simulink model "uplink_4c1r"  (Simulink 8.7)
settings: Solver=VariableStepDiscrete  StartTime=0.0  StopTime=DDC_Lineup_param.endTime  RelTol=1e-3
PreLoadFcn:
  | % Run the setup script when the model is opened
  | setup_uplink_4c1r;
InitFcn:
  | % Run the setup script again just before the
  | % model is run, so that any updates made
  | % after opening are applied.
  | setup_uplink_4c1r;
  | %% DSPBuilder Start
  | alt_dspbuilder_update_model(bdroot)
  | %% DSPBuilder End
undefined symbols (not defined in the file or in its folder): AdvDSPBChannelOutDisplay, carrier_separation, DDC_Lineup_param, dpoly, dspba_ChannelInVis, dspba_ChannelOutVis, dspba_internal_get_channel_ports, dspba_internal_get_demux_ports, evalAionMaskParam, latency, Power_Meter, primtype, Subsystem, uplink_4c1r_carrier_seperation_4c, uplink_4c1r_pd_accu_reg_block, uplink_4c1r_power_meter_1carrier, value
undefined symbols (not defined in the file): power_meter_param
libraries: DSPBAPrim x119, DSPBABase x26, uplink_4c1r_pipereg_lib x22, DSPBAModelBus x9, DSPBAFilters x5, uplink_4c1r_register x5, uplink_4c1r_accumulator x5, uplink_4c1r_peak_detector x5, uplink_4c1r_iq_square x4, DSPBAControl x2, DSPBAWaveformSynth x2, DSPBAUtilities x1
(part 1 of 3)
Description:
  | DSP Builder Advanced Template for Template Design implementing ModelIP designs
settings Model: Creator=mjervis  LastModifiedBy=5g
settings DataIOCC: SignalLoggingSaveFormat=ModelDataLogs
settings OptimizationCC: ExpressionDepthLimit=2147483647
settings DebuggingCC: SolverPrmCheckMsg=warning  InheritedTsInSrcMsg=none  IntegerOverflowMsg=none  FcnCallInpInsideContextMsg=UseLocalSettings  StateNameClashWarn=warning  IntegerSaturationMsg=none
settings GRTTargetCC: CombineOutputUpdateFcns=off  GRTInterface=on

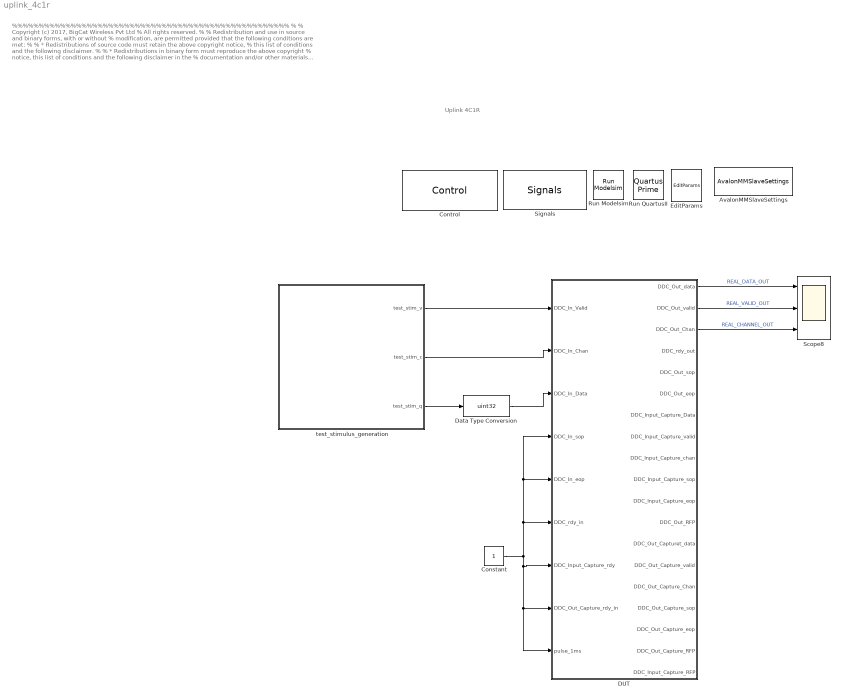
== system uplink_4c1r ==
  note: %%%%%%%%%%%%%%%%%%%%%%%%%%%%%%%%%%%%%%%%%%%%%%%%%%%%
      |  %
      |  % Copyright (c) 2017, BigCat Wireless Pvt Ltd
      |  % All rights reserved.
      |  %
      |  % Redistribution and use in source and binary forms, with or without
      |  % modification, are permitted provided that the following conditions are met:
      |  %
      |  %     * Redistributions of source code must retain the above copyright notice,
      |  %       this list of conditions and the following disclaimer.
      |  %
      |  %     * Redistributions in binary form must reproduce the above copyright
      |  %       notice, this list of conditions and the following disclaimer in the
      |  %       documentation and/or other materials provided with the distribution.
      |  %
      |  %     * Neither the name of the copyright holder nor the names of its contributors
      |  %       may be used to endorse or promote products derived from this software
      |  %       without specific prior written permission.
      |  %
      |  %
      |  %
      |  % THIS SOFTWARE IS PROVIDED BY THE COPYRIGHT HOLDERS AND CONTRIBUTORS "AS IS"
      |  % AND ANY EXPRESS OR IMPLIED WARRANTIES, INCLUDING, BUT NOT LIMITED TO, THE
      |  % IMPLIED WARRANTIES OF MERCHANTABILITY AND FITNESS FOR A PARTICULAR PURPOSE ARE
      |  % DISCLAIMED. IN NO EVENT SHALL THE COPYRIGHT HOLDER OR CONTRIBUTORS BE LIABLE
      |  % FOR ANY DIRECT, INDIRECT, INCIDENTAL, SPECIAL, EXEMPLARY, OR CONSEQUENTIAL
      |  % DAMAGES (INCLUDING, BUT NOT LIMITED TO, PROCUREMENT OF SUBSTITUTE GOODS OR
      |  % SERVICES; LOSS OF USE, DATA, OR PROFITS; OR BUSINESS INTERRUPTION) HOWEVER
      |  % CAUSED AND ON ANY THEORY OF LIABILITY, WHETHER IN CONTRACT, STRICT LIABILITY,
      |  % OR TORT (INCLUDING NEGLIGENCE OR OTHERWISE) ARISING IN ANY WAY OUT OF THE USE
      |  % OF THIS SOFTWARE, EVEN IF ADVISED OF THE POSSIBILITY OF SUCH DAMAGE.
      |  %
      |   %%%%%%%%%%%%%%%%%%%%%%%%%%%%%%%%%%%%%%%%%%%%%%%%%%%%%
  note: Uplink 4C1R
  AvalonMMSlaveSettings : DSPBABase/AvalonMMSlaveSettings
  Constant : Constant  OutDataTypeStr=boolean
  Control : DSPBABase/Control  generate=on  language=VHDL  destination=./rtl  destination_gui=./rtl  make_full_path=off  path_is_relative=on  autotestbench=off  signaldepth=2  coveragetestbench=on  logs=off  spacewidth=2  spacenum=1  addrwidth=10  datawidth=32  dataendian=Big Endian  hierarchicalnames=off  ramThresholdBits=-1  distRamThresholdBits=-1  mlabThresholdBits=-1  hardMultiplierThresholdLuts=-1  version=20090407  errorOnChanMismatch=1  errorOnGPIOMismatch=0  importModelsimResults=0  cycleAccurate=off  reinterpretCastMult=off  paramFile=uplink_4c1r_params.xml
  DUT : Subsystem
  Data Type Conversion : DataTypeConversion  OutDataTypeStr=uint32
  EditParams : DSPBABase/EditParams  version=20090407
  Run Modelsim : DSPBABase/Run Modelsim  version=20090407
  "Run QuartusII " : DSPBABase/Quartus Prime  version=20090407
  Scope8 : Scope  NumInputPorts=3
  Signals : DSPBABase/Signals  clk=clk  freq=DDC_Lineup_param.ClockRate  margin=DDC_Lineup_param.ClockMargin  rst=areset  rstactive=High  bus=bus  enbusclock=on  busfreq=DDC_Lineup_param.ClockRate/10  bussync=on  version=20090407
  test_stimulus_generation : Subsystem
  wires:
  test_stimulus_generation/3(test_stim_q) -> Data Type Conversion/1
  DUT/1(DDC_Out_data) -> Scope8/1  "REAL_DATA_OUT"
  Constant/1 -> DUT/7(DDC_Input_Capture_rdy), DUT/8(DDC_Out_Capture_rdy_in), DUT/9(pulse_1ms), DUT/5(DDC_In_eop), DUT/4(DDC_In_sop), DUT/6(DDC_rdy_in)
  Data Type Conversion/1 -> DUT/3(DDC_In_Data)
  test_stimulus_generation/2(test_stim_c) -> DUT/2(DDC_In_Chan)
  test_stimulus_generation/1(test_stim_v) -> DUT/1(DDC_In_Valid)
  DUT/2(DDC_Out_valid) -> Scope8/2  "REAL_VALID_OUT"
  DUT/3(DDC_Out_Chan) -> Scope8/3  "REAL_CHANNEL_OUT"

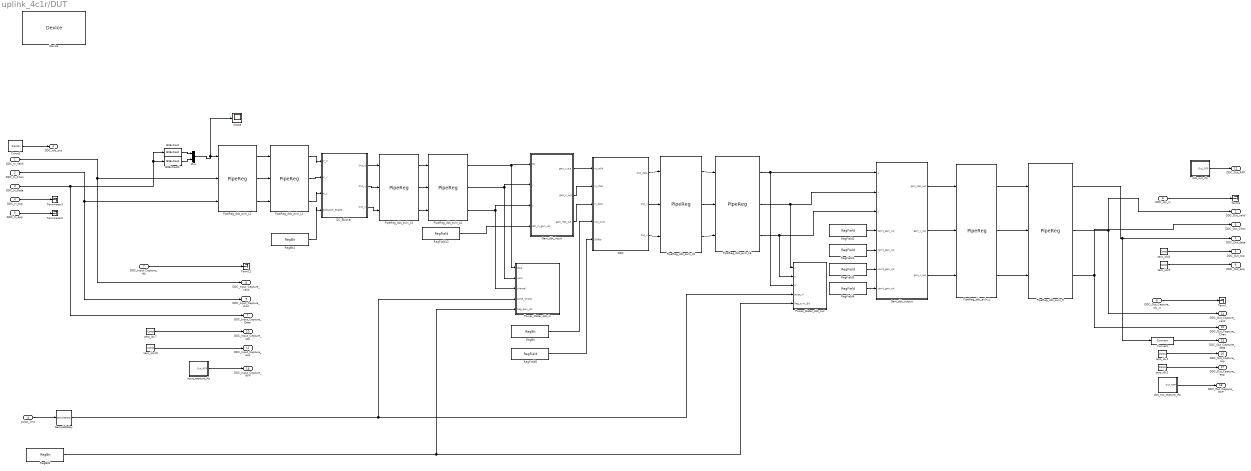
== system uplink_4c1r/DUT ==
  DDC_In_Valid : Inport
  DDC_In_Chan : Inport  Port=2
  DDC_In_Data : Inport  Port=3
  DDC_In_sop : Inport  Port=4  OutDataTypeStr=boolean
  DDC_In_eop : Inport  Port=5  OutDataTypeStr=boolean
  DDC_rdy_in : Inport  Port=6  OutDataTypeStr=boolean
  DDC_Input_Capture_rdy : Inport  Port=7  OutDataTypeStr=boolean
  DDC_Out_Capture_rdy_in : Inport  Port=8  OutDataTypeStr=boolean
  pulse_1ms : Inport  Port=9
  BitExtract : DSPBAPrim/BitExtract  primtype=bitextract  nInputs=1  nOutputs=1  omode=Specify via dialog  otype=sfix(16)  scale=2^-15  rndmethod=Unbiased  factor=1  satmethod=Symmetric  shift_vec=[0 1 2 -1]  value=0  inPortNames=[' '; ' ';]  outPortNames=[' ']  dspbaimage=dspba_prim.jpg  text=fprintf('..%d', value);  style=Optimised  visibilities=8+1024  version=20090407
  BitExtract1 : DSPBAPrim/BitExtract  primtype=bitextract  nInputs=1  nOutputs=1  omode=Specify via dialog  otype=sfix(16)  scale=2^-15  rndmethod=Unbiased  factor=1  satmethod=Symmetric  shift_vec=[0 1 2 -1]  value=16  inPortNames=[' '; ' ';]  outPortNames=[' ']  dspbaimage=dspba_prim.jpg  text=fprintf('..%d', value);  style=Optimised  visibilities=8+1024  version=20090407
  Const2 : DSPBAPrim/Const  primtype=const  nInputs=0  nOutputs=1  omode=boolean  otype=sfix(16)  scale=2^-15  rndmethod=Unbiased  factor=1  satmethod=Symmetric  shift_vec=[0 1 2 -1]  value=1  inPortNames=['+'; '+';]  outPortNames=[' ']  dspbaimage=dspba_prim.jpg  text=fprintf('%s', num2str(value));  style=Optimised  visibilities=8 + 1024  floatPrecision=float32_m23  version=20120820
  Convert : DSPBAPrim/Convert  primtype=convert  nInputs=1  nOutputs=1  omode=Specify via dialog  otype=sfix(32)  scale=2^-31  rndmethod=Unbiased  factor=1  satmethod=None  shift_vec=[0 1 2 -1]  value=round([0:255]/17)  inPortNames=[' '; ' ';]  outPortNames=[' '; 'c']  dspbaimage=dspba_prim.jpg  text=fprintf('convert');  style=Optimised  visibilities=8+64+256+2^17  clipdetect=off  floatPrecision=float32_m23  advOptions=[]  version=20130211
  DC_Blocker : Subsystem
  DDC : Subsystem
  Device : DSPBABase/Device  family=Arria 10  deviceMember=Arria 10  stratix4device=Stratix IV GX  hardcopy4device=HardCopy IV E  stratix5device=Stratix V GX  device=10AS066N3F40E2SGE2  speed=2  stratixSpeed=-5  stratix2Speed=-3  stratix3Speed=-3  stratix4gxSpeed=-2  stratix4gtSpeed=-1  cyclone2Speed=-6  cyclone3Speed=-7  arria2Speed=-4  cyclone4eSpeed=-8  stratix5Speed=-3  arria5Speed=-4  arriaSpeed=-6  cyclone3lsSpeed=-7  cyclone5Speed=-6  arria2gzSpeed=-3  nightFurySpeed=-2  ecp2Speed=-7  hardcopycompat=off  version=20140217  max10flashmode=off  max10nomeminit=off
  Gain_ddc_input : Subsystem
  Gain_ddc_output : Subsystem
  Mux : Mux  Inputs=2
  PipeReg_ddc_avln_L : uplink_4c1r_pipereg_lib/PipeReg  NPipe=2  Clock_Margin=100
      link override ChannelOut: latency=2
  PipeReg_ddc_avln_L1 : uplink_4c1r_pipereg_lib/PipeReg  NPipe=2  Clock_Margin=100
      link override ChannelOut: latency=2
  PipeReg_ddc_avln_L2 : uplink_4c1r_pipereg_lib/PipeReg  NPipe=2  Clock_Margin=100
      link override ChannelOut: latency=2
  PipeReg_ddc_avln_L3 : uplink_4c1r_pipereg_lib/PipeReg  NPipe=2  Clock_Margin=100
      link override ChannelOut: latency=2
  PipeReg_ddc_avln_L4 : uplink_4c1r_pipereg_lib/PipeReg  NPipe=2  Clock_Margin=100
      link override ChannelOut: latency=2
  PipeReg_ddc_avln_L5 : uplink_4c1r_pipereg_lib/PipeReg  NPipe=2  Clock_Margin=100
      link override ChannelOut: latency=2
  PipeReg_ddc_avln_L6 : uplink_4c1r_pipereg_lib/PipeReg  NPipe=2  Clock_Margin=100
      link override ChannelOut: latency=2
  PipeReg_ddc_avln_R : uplink_4c1r_pipereg_lib/PipeReg  NPipe=2  Clock_Margin=100
      link override ChannelOut: latency=2
  Power_Meter_ddc_in : Subsystem  AncestorBlock=uplink_4c1r_power_meter_1carrier/Power_Meter  mask{Latency=20, Peak_Detector_address=power_meter_param.ddc_in_pd_address, Accumulator1_addr=power_meter_param.ddc1_in_acc1_reg_addr, Accumulator2_addr=power_meter_param.ddc1_in_acc2_reg_addr}
      mask Display:
      | disp('Power_Meter');
      | port_label('input',1,'d');
      | port_label('input',2,'v');
      | port_label('input',3,'c');
      | port_label('input',4,'pulse_in');
      | port_label('input',5,'Reg_busy_bit');
  Power_Meter_ddc_out : Subsystem
  RegBit : DSPBAModelBus/RegBit  reg_name=DDC_LINEUP_param.NCO.Sync  reg_rwmode=Read/Write  reg_lsb=1  reg_init=0  reg_desc=NCO_SYNC_BIT  reg_addr=512  reg_desc0=0  reg_desc1=0  SampleTime=1  version=20090407
  RegBit1 : DSPBAModelBus/RegBit  reg_name=DDC_LINEUP_param.DC_Blocker_En  reg_rwmode=Read/Write  reg_lsb=1  reg_init=DC_Blocker_Initial_Value  reg_desc=To Enable DC Blocker  reg_addr=912  reg_desc0=0  reg_desc1=0  SampleTime=1  version=20090407
  RegBit2 : DSPBAModelBus/RegBit  reg_name=Reg_busy_bit_addr  reg_rwmode=Read/Write  reg_lsb=0  reg_init=0  reg_desc=Reg_busy_bi will be stored here  reg_addr=933  reg_desc0=0  reg_desc1=0  SampleTime=-1  version=20090407
  RegField1 : DSPBAModelBus/RegField  reg_name=carr2_gain_addr  reg_rwmode=Read/Write  reg_msb=15  reg_lsb=0  reg_mode=Specify via dialog  reg_type=ufix(16)  reg_scale=2^-12  reg_init=carr2_gain_val_init  reg_desc=carr2_gain will be stored here  reg_modal=off  reg_desc0=0  reg_desc1=0  reg_desc2=0  reg_desc3=0  reg_desc4=0  reg_desc5=0  reg_desc6=0  reg_desc7=0  reg_addr=915  SampleTime=-1  version=20090407
  RegField12 : DSPBAModelBus/RegField  reg_name=ddc_in_gain_addr  reg_rwmode=Read/Write  reg_msb=15  reg_lsb=0  reg_mode=Specify via dialog  reg_type=ufix(16)  reg_scale=2^-12  reg_init=ddc_in_gain_init_value  reg_desc=ddc_in_gain_init_value will be stored here  reg_modal=off  reg_desc0=0  reg_desc1=0  reg_desc2=0  reg_desc3=0  reg_desc4=0  reg_desc5=0  reg_desc6=0  reg_desc7=0  reg_addr=913  SampleTime=-1  version=20090407
  RegField2 : DSPBAModelBus/RegField  reg_name=carr1_gain_addr  reg_rwmode=Read/Write  reg_msb=15  reg_lsb=0  reg_mode=Specify via dialog  reg_type=ufix(16)  reg_scale=2^-12  reg_init=carr1_gain_val_init  reg_desc=carr1_gain will be stored here  reg_modal=off  reg_desc0=0  reg_desc1=0  reg_desc2=0  reg_desc3=0  reg_desc4=0  reg_desc5=0  reg_desc6=0  reg_desc7=0  reg_addr=914  SampleTime=-1  version=20090407
  RegField3 : DSPBAModelBus/RegField  reg_name=carr3_gain_addr  reg_rwmode=Read/Write  reg_msb=15  reg_lsb=0  reg_mode=Specify via dialog  reg_type=ufix(16)  reg_scale=2^-12  reg_init=carr3_gain_val_init  reg_desc=carr3_gain will be stored here  reg_modal=off  reg_desc0=0  reg_desc1=0  reg_desc2=0  reg_desc3=0  reg_desc4=0  reg_desc5=0  reg_desc6=0  reg_desc7=0  reg_addr=916  SampleTime=-1  version=20090407
  RegField4 : DSPBAModelBus/RegField  reg_name=carr4_gain_addr  reg_rwmode=Read/Write  reg_msb=15  reg_lsb=0  reg_mode=Specify via dialog  reg_type=ufix(16)  reg_scale=2^-12  reg_init=carr4_gain_val_init  reg_desc=carr4_gain will be stored here  reg_modal=off  reg_desc0=0  reg_desc1=0  reg_desc2=0  reg_desc3=0  reg_desc4=0  reg_desc5=0  reg_desc6=0  reg_desc7=0  reg_addr=917  SampleTime=-1  version=20090407
  RegField5 : DSPBAModelBus/RegField  reg_name=Shifter_Bits  reg_rwmode=Read/Write  reg_msb=1  reg_lsb=0  reg_mode=Specify via dialog  reg_type=ufix(2)  reg_scale=2^-0  reg_init=Mixer_Shifter_init_value  reg_desc=ddc_in_gain_init_value will be stored here  reg_modal=off  reg_desc0=0  reg_desc1=0  reg_desc2=0  reg_desc3=0  reg_desc4=0  reg_desc5=0  reg_desc6=0  reg_desc7=0  reg_addr=934  SampleTime=-1  version=20090407
  SampleDelay : DSPBAPrim/SampleDelay  primtype=sampdelay  nInputs=1  nOutputs=1  omode=Inherit via internal rule  otype=sfix(16)  scale=2^-15  rndmethod=Unbiased  factor=1  satmethod=Symmetric  shift_vec=[0 1 2 -1]  value=4  inPortNames=[' '; ' ';]  outPortNames=[' ']  dspbaimage=dspba_prim.jpg  text=dpoly(1, eye(1,value+1), 'z')  style=Optimised  visibilities=8 + 1024 + 2^17 + 2^18  flexible=off  slackgroup=0  augmented=0  version=20090407  advOptions=[]
  Scope : Scope
  Term1 : Terminator
  Term12 : Terminator
  Term6 : Terminator
  Terminator1 : Terminator
  Terminator2 : Terminator
  ddc_out_capture_rfp : Subsystem
  ddc_out_rfp : Subsystem
  input_capture_rfp : Subsystem
  zero_idx{1..2,8..9} (4 alike) : DSPBAPrim/Const  primtype=const  nInputs=0  nOutputs=1  omode=Specify via dialog  otype=ufix(1)  scale=0  rndmethod=Unbiased  factor=1  satmethod=Symmetric  shift_vec=[0 1 2 -1]  value=0  inPortNames=['+'; '+';]  outPortNames=[' ']  dspbaimage=dspba_prim.jpg  text=fprintf('%s', num2str(value));  style=Optimised  visibilities=8 + 1024  floatPrecision=float32_m23  version=20120820
  zero_idx10 : DSPBAPrim/Const  primtype=const  nInputs=0  nOutputs=1  omode=boolean  otype=ufix(1)  scale=0  rndmethod=Unbiased  factor=1  satmethod=Symmetric  shift_vec=[0 1 2 -1]  value=0  inPortNames=['+'; '+';]  outPortNames=[' ']  dspbaimage=dspba_prim.jpg  text=fprintf('%s', num2str(value));  style=Optimised  visibilities=8 + 1024  floatPrecision=float32_m23  version=20120820
  zero_idx7 : DSPBAPrim/Const  primtype=const  nInputs=0  nOutputs=1  omode=boolean  otype=ufix(1)  scale=0  rndmethod=Unbiased  factor=1  satmethod=Symmetric  shift_vec=[0 1 2 -1]  value=0  inPortNames=['+'; '+';]  outPortNames=[' ']  dspbaimage=dspba_prim.jpg  text=fprintf('%s', num2str(value));  style=Optimised  visibilities=8 + 1024  floatPrecision=float32_m23  version=20120820
  DDC_Out_data : Outport
  DDC_Out_valid : Outport  Port=2
  DDC_Out_Chan : Outport  Port=3
  DDC_rdy_out : Outport  Port=4
  DDC_Out_sop : Outport  Port=5
  DDC_Out_eop : Outport  Port=6
  DDC_Input_Capture_Data : Outport  Port=7
  DDC_Input_Capture_valid : Outport  Port=8
  DDC_Input_Capture_chan : Outport  Port=9
  DDC_Input_Capture_sop : Outport  Port=10
  DDC_Input_Capture_eop : Outport  Port=11
  DDC_Out_RFP : Outport  Port=12
  DDC_Out_Capturet_data : Outport  Port=13
  DDC_Out_Capture_valid : Outport  Port=14
  DDC_Out_Capture_Chan : Outport  Port=15
  DDC_Out_Capture_sop : Outport  Port=16
  DDC_Out_Capture_eop : Outport  Port=17
  DDC_Out_Capture_RFP : Outport  Port=18
  DDC_Input_Capture_RFP : Outport  Port=19
  wires:
  DDC_In_sop/1 -> Terminator1/1
  DDC_In_eop/1 -> Terminator2/1
  Const2/1 -> DDC_rdy_out/1
  DDC_rdy_in/1 -> Term6/1
  zero_idx8/1 -> DDC_Out_sop/1
  zero_idx9/1 -> DDC_Out_eop/1
  DDC_In_Data/1 -> DDC_Input_Capture_Data/1, BitExtract1/1, BitExtract/1
  DDC_In_Chan/1 -> PipeReg_ddc_avln_L2/3, DDC_Input_Capture_chan/1
  DDC_Input_Capture_rdy/1 -> Term12/1
  zero_idx7/1 -> DDC_Input_Capture_sop/1
  zero_idx10/1 -> DDC_Input_Capture_eop/1
  ddc_out_rfp/1(Out_RFP) -> DDC_Out_RFP/1
  Convert/1 -> DDC_Out_Capturet_data/1
  DDC_Out_Capture_rdy_in/1 -> Term1/1
  zero_idx1/1 -> DDC_Out_Capture_sop/1
  zero_idx2/1 -> DDC_Out_Capture_eop/1
  ddc_out_capture_rfp/1(Out_RFP) -> DDC_Out_Capture_RFP/1
  input_capture_rfp/1(Out_RFP) -> DDC_Input_Capture_RFP/1
  RegBit/1 -> DDC/4(nco_sync)
  PipeReg_ddc_avln_L/3 -> PipeReg_ddc_avln_R/3
  PipeReg_ddc_avln_L/2 -> PipeReg_ddc_avln_R/2
  PipeReg_ddc_avln_L/1 -> PipeReg_ddc_avln_R/1
  DDC_In_Valid/1 -> PipeReg_ddc_avln_L2/2, DDC_Input_Capture_valid/1
  BitExtract/1 -> Mux/1
  BitExtract1/1 -> Mux/2
  PipeReg_ddc_avln_R/1 -> Convert/1, DDC_Out_data/1
  PipeReg_ddc_avln_R/2 -> DDC_Out_valid/1, DDC_Out_Capture_valid/1
  PipeReg_ddc_avln_R/3 -> DDC_Out_Chan/1, DDC_Out_Capture_Chan/1
  RegBit1/1 -> DC_Blocker/4(dcblocker_Enable)
  PipeReg_ddc_avln_L1/1 -> DC_Blocker/1(In_d)
  PipeReg_ddc_avln_L1/2 -> DC_Blocker/2(In_v)
  PipeReg_ddc_avln_L1/3 -> DC_Blocker/3(In_c)
  PipeReg_ddc_avln_L2/1 -> PipeReg_ddc_avln_L1/1
  PipeReg_ddc_avln_L2/2 -> PipeReg_ddc_avln_L1/2
  PipeReg_ddc_avln_L2/3 -> PipeReg_ddc_avln_L1/3
  RegField12/1 -> Gain_ddc_input/4(ddc_in_gain_val)
  DC_Blocker/1(Out_q) -> PipeReg_ddc_avln_L3/1
  DC_Blocker/2(Out_v) -> PipeReg_ddc_avln_L3/2
  DC_Blocker/3(Out_c) -> PipeReg_ddc_avln_L3/3
  PipeReg_ddc_avln_L3/1 -> PipeReg_ddc_avln_L4/1
  PipeReg_ddc_avln_L3/3 -> PipeReg_ddc_avln_L4/3
  PipeReg_ddc_avln_L3/2 -> PipeReg_ddc_avln_L4/2
  PipeReg_ddc_avln_L4/1 -> Power_Meter_ddc_in/1("data "), Gain_ddc_input/1(d0)
  PipeReg_ddc_avln_L4/2 -> Power_Meter_ddc_in/2(valid), Gain_ddc_input/2(v)
  PipeReg_ddc_avln_L4/3 -> Power_Meter_ddc_in/3(channel), Gain_ddc_input/3(c)
  Mux/1 -> Scope/1, PipeReg_ddc_avln_L2/1
  Gain_ddc_input/1(gain_v_out) -> DDC/1(In_valid)
  Gain_ddc_input/2(gain_c_out) -> DDC/2(In_chan)
  Gain_ddc_input/3(gain_real_out) -> DDC/3(In_data)
  RegField2/1 -> Gain_ddc_output/4(carr1_gain_val)
  RegField1/1 -> Gain_ddc_output/5(carr2_gain_val)
  RegField3/1 -> Gain_ddc_output/6(carr3_gain_val)
  RegField4/1 -> Gain_ddc_output/7(carr4_gain_val)
  Gain_ddc_output/1(gain_real_out) -> PipeReg_ddc_avln_L/1
  Gain_ddc_output/2(gain_v_out) -> PipeReg_ddc_avln_L/2
  Gain_ddc_output/3(gain_c_out) -> PipeReg_ddc_avln_L/3
  DDC/1(Out_data) -> PipeReg_ddc_avln_L5/1
  DDC/2(Out_v) -> PipeReg_ddc_avln_L5/2
  DDC/3(Out_c) -> PipeReg_ddc_avln_L5/3
  PipeReg_ddc_avln_L5/2 -> PipeReg_ddc_avln_L6/2
  PipeReg_ddc_avln_L6/1 -> Power_Meter_ddc_out/3(d), Gain_ddc_output/1(a)
  PipeReg_ddc_avln_L6/2 -> Power_Meter_ddc_out/1(v), Gain_ddc_output/2(v)
  PipeReg_ddc_avln_L6/3 -> Gain_ddc_output/3(c), Power_Meter_ddc_out/2(c)
  pulse_1ms/1 -> SampleDelay/1
  SampleDelay/1 -> Power_Meter_ddc_in/4(pulse_1msec), Power_Meter_ddc_out/4(pulse_in)
  RegBit2/1 -> Power_Meter_ddc_out/5(Reg_sync_Bit), Power_Meter_ddc_in/5(Reg_busy_bit)
  RegField5/1 -> DDC/5(Shifter)
  PipeReg_ddc_avln_L5/1 -> PipeReg_ddc_avln_L6/1
  PipeReg_ddc_avln_L5/3 -> PipeReg_ddc_avln_L6/3

== system uplink_4c1r/test_stimulus_generation ==
  Create Channelized  Input Data1 : DSPBAUtilities/Channelizer  data_input=DDC_Lineup_param.inputdata1  folding=DDC_Lineup_param.Period  samples_valid=1  samples_idle=0  sample_time=1
  test_stim_v : Outport
  test_stim_c : Outport  Port=2
  test_stim_q : Outport  Port=3
  wires:
  Create Channelized  Input Data1/1 -> test_stim_q/1
  Create Channelized  Input Data1/2 -> test_stim_v/1
  Create Channelized  Input Data1/3 -> test_stim_c/1

== system uplink_4c1r/DUT/DC_Blocker ==
  In_d : Inport
  In_v : Inport  Port=2
  In_c : Inport  Port=3
  dcblocker_Enable : Inport  Port=4
  Scale : DSPBABase/Scale  otype=sfix(16)  scale=2^-15  rndmethod=Unbiased  factor=1  satmethod=Symmetric  shift_vec=-8  latency=6  wideSimulation=off  version=20130807
  Terminator3 : Terminator
  accumulator : Subsystem
  mean_sub : Subsystem
  zero_idx1 : DSPBAPrim/Const  primtype=const  nInputs=0  nOutputs=1  omode=Inherit via internal rule  otype=sfix(16)  scale=2^-15  rndmethod=Unbiased  factor=1  satmethod=Symmetric  shift_vec=[0 1 2 -1]  value=0  inPortNames=['+'; '+';]  outPortNames=[' ']  dspbaimage=dspba_prim.jpg  text=fprintf('%s', num2str(value));  style=Optimised  visibilities=8 + 1024  floatPrecision=float32_m23  version=20120820
  Out_q : Outport
  Out_v : Outport  Port=2
  Out_c : Outport  Port=3
  wires:
  mean_sub/3(dcblocker_meansub_q_out) -> Out_q/1
  mean_sub/1(dcblocker_meansub_v_out) -> Out_v/1
  In_v/1 -> accumulator/1(dcblocker_acc_v_in), mean_sub/2(dcblocker_data_v_in)
  In_d/1 -> accumulator/3(dcblocker_acc_q_in), mean_sub/1(dcblocker_data_q_in)
  In_c/1 -> accumulator/2(dcblocker_acc_c_in), mean_sub/3(dcblocker_data_c_in)
  accumulator/1(dcblocker_acc_q_out) -> Scale/1
  accumulator/2(dcblocker_acc_v_out) -> Scale/2
  accumulator/3(dcblocker_acc_c_out) -> Scale/3
  Scale/4 -> Terminator3/1
  zero_idx1/1 -> Scale/4
  Scale/1 -> mean_sub/4(dcblocker_mean_q_in)
  Scale/2 -> mean_sub/5(dcblocker_mean_v_in)
  Scale/3 -> mean_sub/6(dcblocker_mean_c_in)
  mean_sub/2(dcblocker_meansub_c_out) -> Out_c/1
  dcblocker_Enable/1 -> mean_sub/7(dcblocker_Enable)

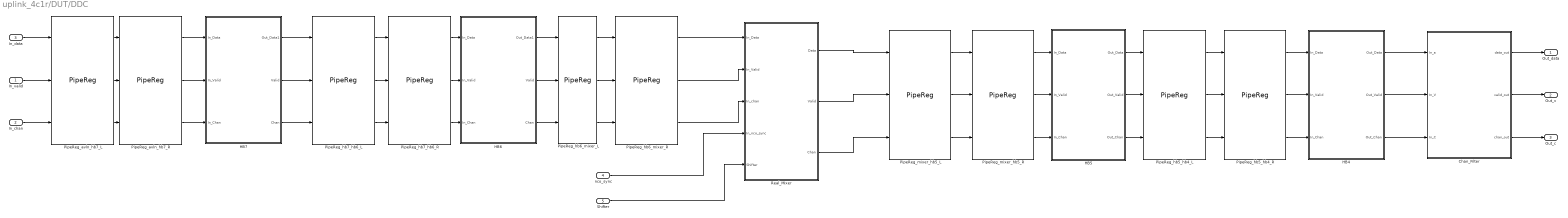
== system uplink_4c1r/DUT/DDC ==
  In_valid : Inport
  In_chan : Inport  Port=2
  In_data : Inport  Port=3
  nco_sync : Inport  Port=4
  Shifter : Inport  Port=5
  Chan_Filter : Subsystem
  HB4 : Subsystem
  HB5 : Subsystem
  HB6 : Subsystem
  HB7 : Subsystem
  PipeReg_avln_hb7_L : uplink_4c1r_pipereg_lib/PipeReg  NPipe=2  Clock_Margin=100
      link override ChannelOut: value=1  packetBeginEnabled=off  latency=2
  PipeReg_avln_hb7_R : uplink_4c1r_pipereg_lib/PipeReg  NPipe=2  Clock_Margin=100
      link override ChannelOut: value=1  packetBeginEnabled=off  latency=2
  PipeReg_hb5_hb4_L : uplink_4c1r_pipereg_lib/PipeReg  NPipe=2  Clock_Margin=100
      link override ChannelOut: value=1  packetBeginEnabled=off  latency=2
  PipeReg_hb5_hb4_R : uplink_4c1r_pipereg_lib/PipeReg  NPipe=2  Clock_Margin=100
      link override ChannelOut: value=1  packetBeginEnabled=off  latency=2
  PipeReg_hb6_mixer_L : uplink_4c1r_pipereg_lib/PipeReg  NPipe=2  Clock_Margin=100
      link override ChannelOut: value=1  packetBeginEnabled=off  latency=2
  PipeReg_hb6_mixer_R : uplink_4c1r_pipereg_lib/PipeReg  NPipe=2  Clock_Margin=100
      link override ChannelOut: value=1  packetBeginEnabled=off  latency=2
  PipeReg_hb7_hb6_L : uplink_4c1r_pipereg_lib/PipeReg  NPipe=2  Clock_Margin=100
      link override ChannelOut: value=1  packetBeginEnabled=off  latency=2
  PipeReg_hb7_hb6_R : uplink_4c1r_pipereg_lib/PipeReg  NPipe=2  Clock_Margin=100
      link override ChannelOut: value=1  packetBeginEnabled=off  latency=2
  PipeReg_mixer_hb5_L : uplink_4c1r_pipereg_lib/PipeReg  NPipe=2  Clock_Margin=100
      link override ChannelOut: value=1  packetBeginEnabled=off  latency=2
  PipeReg_mixer_hb5_R : uplink_4c1r_pipereg_lib/PipeReg  NPipe=2  Clock_Margin=100
      link override ChannelOut: value=1  packetBeginEnabled=off  latency=2
  Real_Mixer : Subsystem
  Out_data : Outport
  Out_v : Outport  Port=2
  Out_c : Outport  Port=3
  wires:
  Chan_Filter/1(data_out) -> Out_data/1
  Chan_Filter/2(valid_out) -> Out_v/1
  Chan_Filter/3(chan_out) -> Out_c/1
  nco_sync/1 -> Real_Mixer/4(In_nco_sync)
  HB4/1(Out_Data) -> Chan_Filter/1(In_a)
  HB4/2(Out_Valid) -> Chan_Filter/2(In_V)
  HB4/3(Out_Chan) -> Chan_Filter/3(In_C)
  HB7/1(Out_Data1) -> PipeReg_hb7_hb6_L/1
  HB7/3(Chan) -> PipeReg_hb7_hb6_L/3
  PipeReg_hb7_hb6_L/2 -> PipeReg_hb7_hb6_R/2
  PipeReg_hb7_hb6_L/3 -> PipeReg_hb7_hb6_R/3
  PipeReg_hb7_hb6_L/1 -> PipeReg_hb7_hb6_R/1
  PipeReg_hb7_hb6_R/3 -> HB6/3(In_Chan)
  PipeReg_hb7_hb6_R/1 -> HB6/1(In_Data)
  PipeReg_hb7_hb6_R/2 -> HB6/2(In_Valid)
  HB6/1(Out_Data1) -> PipeReg_hb6_mixer_L/1
  HB6/2(Valid) -> PipeReg_hb6_mixer_L/2
  HB6/3(Chan) -> PipeReg_hb6_mixer_L/3
  PipeReg_hb6_mixer_L/2 -> PipeReg_hb6_mixer_R/2
  PipeReg_hb6_mixer_L/3 -> PipeReg_hb6_mixer_R/3
  PipeReg_hb6_mixer_L/1 -> PipeReg_hb6_mixer_R/1
  PipeReg_hb6_mixer_R/1 -> Real_Mixer/1(In_Data)
  PipeReg_hb6_mixer_R/2 -> Real_Mixer/2("In_Valid ")
  PipeReg_hb6_mixer_R/3 -> Real_Mixer/3("In_chan ")
  Real_Mixer/1(Data) -> PipeReg_mixer_hb5_L/1
  Real_Mixer/2(Valid) -> PipeReg_mixer_hb5_L/2
  Real_Mixer/3(Chan) -> PipeReg_mixer_hb5_L/3
  PipeReg_mixer_hb5_L/1 -> PipeReg_mixer_hb5_R/1
  PipeReg_mixer_hb5_L/2 -> PipeReg_mixer_hb5_R/2
  PipeReg_mixer_hb5_L/3 -> PipeReg_mixer_hb5_R/3
  PipeReg_mixer_hb5_R/1 -> HB5/1(In_Data)
  PipeReg_mixer_hb5_R/2 -> HB5/2(In_Valid)
  PipeReg_mixer_hb5_R/3 -> HB5/3(In_Chan)
  HB5/2(Out_Valid) -> PipeReg_hb5_hb4_L/2
  HB5/3(Out_Chan) -> PipeReg_hb5_hb4_L/3
  HB5/1(Out_Data) -> PipeReg_hb5_hb4_L/1
  PipeReg_hb5_hb4_L/1 -> PipeReg_hb5_hb4_R/1
  PipeReg_hb5_hb4_L/2 -> PipeReg_hb5_hb4_R/2
  PipeReg_hb5_hb4_L/3 -> PipeReg_hb5_hb4_R/3
  PipeReg_hb5_hb4_R/1 -> HB4/1(In_Data)
  PipeReg_hb5_hb4_R/2 -> HB4/2(In_Valid)
  PipeReg_hb5_hb4_R/3 -> HB4/3(In_Chan)
  PipeReg_avln_hb7_L/2 -> PipeReg_avln_hb7_R/2
  PipeReg_avln_hb7_L/3 -> PipeReg_avln_hb7_R/3
  PipeReg_avln_hb7_L/1 -> PipeReg_avln_hb7_R/1
  In_chan/1 -> PipeReg_avln_hb7_L/3
  In_valid/1 -> PipeReg_avln_hb7_L/2
  In_data/1 -> PipeReg_avln_hb7_L/1
  PipeReg_avln_hb7_R/3 -> HB7/3(In_Chan)
  HB7/2(Valid) -> PipeReg_hb7_hb6_L/2
  PipeReg_avln_hb7_R/1 -> HB7/1(In_Data)
  PipeReg_avln_hb7_R/2 -> HB7/2(In_Valid)
  Shifter/1 -> Real_Mixer/5(Shifter)

== system uplink_4c1r/DUT/Gain_ddc_input ==
  d0 : Inport
  v : Inport  Port=2
  c : Inport  Port=3
  ddc_in_gain_val : Inport  Port=4
  Demux : Demux  Outputs=2
  Mux : Mux  Inputs=2
  Subsystem : Subsystem
  Term : Terminator
  scale_gain : DSPBABase/Scale  otype=sfix(16 )  scale=2^-15  rndmethod=Unbiased  factor=1  satmethod=Symmetric  shift_vec=0  latency=7  wideSimulation=off  version=20090407
  zero_idx : DSPBAPrim/Const  primtype=const  nInputs=0  nOutputs=1  omode=Inherit via internal rule  otype=sfix(16)  scale=2^-15  rndmethod=Unbiased  factor=1  satmethod=Symmetric  shift_vec=[0 1 2 -1]  value=0  inPortNames=['+'; '+';]  outPortNames=[' ']  dspbaimage=dspba_prim.jpg  text=fprintf('%s', num2str(value));  style=Optimised  visibilities=8 + 1024  floatPrecision=float32_m23  version=20120820
  gain_v_out : Outport
  gain_c_out : Outport  Port=2
  gain_real_out : Outport  Port=3
  wires:
  ddc_in_gain_val/1 -> Subsystem/5(ddc_in_gain_val)
  scale_gain/3 -> gain_c_out/1
  scale_gain/2 -> gain_v_out/1
  scale_gain/1 -> gain_real_out/1
  Subsystem/2(gain_c_out) -> scale_gain/3
  Subsystem/1(gain_v_out) -> scale_gain/2
  zero_idx/1 -> scale_gain/4
  scale_gain/4 -> Term/1
  c/1 -> Subsystem/4(c)
  v/1 -> Subsystem/3(v)
  Subsystem/3(gain_real_out) -> Mux/1
  Subsystem/4(gain_img_out) -> Mux/2
  Mux/1 -> scale_gain/1
  Demux/1 -> Subsystem/1(d0)
  Demux/2 -> Subsystem/2(d1)
  d0/1 -> Demux/1

== system uplink_4c1r/DUT/Gain_ddc_output ==
  a : Inport
  v : Inport  Port=2
  c : Inport  Port=3
  carr1_gain_val : Inport  Port=4
  carr2_gain_val : Inport  Port=5
  carr3_gain_val : Inport  Port=6
  carr4_gain_val : Inport  Port=7
  Term : Terminator
  gain : Subsystem
  scale_gain : DSPBABase/Scale  otype=sfix(16 )  scale=2^-15  rndmethod=Unbiased  factor=1  satmethod=Symmetric  shift_vec=0  latency=7  wideSimulation=off  version=20090407
  zero_idx : DSPBAPrim/Const  primtype=const  nInputs=0  nOutputs=1  omode=Inherit via internal rule  otype=sfix(16)  scale=2^-15  rndmethod=Unbiased  factor=1  satmethod=Symmetric  shift_vec=[0 1 2 -1]  value=0  inPortNames=['+'; '+';]  outPortNames=[' ']  dspbaimage=dspba_prim.jpg  text=fprintf('%s', num2str(value));  style=Optimised  visibilities=8 + 1024  floatPrecision=float32_m23  version=20120820
  gain_real_out : Outport
  gain_v_out : Outport  Port=2
  gain_c_out : Outport  Port=3
  wires:
  a/1 -> gain/1(a)
  v/1 -> gain/2(v)
  c/1 -> gain/3(c)
  scale_gain/4 -> Term/1
  zero_idx/1 -> scale_gain/4
  gain/1(gain_v_out) -> scale_gain/2
  gain/2(gain_c_out) -> scale_gain/3
  gain/3(gain_real_out) -> scale_gain/1
  scale_gain/1 -> gain_real_out/1
  scale_gain/2 -> gain_v_out/1
  scale_gain/3 -> gain_c_out/1
  carr1_gain_val/1 -> gain/4(carr1_gain_val)
  carr2_gain_val/1 -> gain/5(carr2_gain_val)
  carr4_gain_val/1 -> gain/7(carr4_gain_val)
  carr3_gain_val/1 -> gain/6(carr3_gain_val)

== system uplink_4c1r/DUT/Power_Meter_ddc_in ==
  note: I^2 + Q^2
  "data " : Inport
  valid : Inport  Port=2
  channel : Inport  Port=3
  pulse_1msec : Inport  Port=4
  Reg_busy_bit : Inport  Port=5
  Const : DSPBAPrim/Const  primtype=const  nInputs=0  nOutputs=1  omode=Inherit via internal rule  otype=sfix(16)  scale=2^-15  rndmethod=Unbiased  factor=1  satmethod=Symmetric  shift_vec=[0 1 2 -1]  value=0  inPortNames=['+'; '+';]  outPortNames=[' ']  dspbaimage=dspba_prim.jpg  text=fprintf('%s', num2str(value));  style=Optimised  visibilities=8 + 1024  floatPrecision=float32_m23  version=20120820
  Reg_Block : uplink_4c1r_register/Reg_Block  Peak_Detector_address=13  Accumulator1_addr=14  Accumulator2_addr=15
  Scale : DSPBABase/Scale  otype=sfix(16)  scale=2^-15  rndmethod=Unbiased  factor=1  satmethod=Symmetric  shift_vec=0  latency=6  wideSimulation=off  version=20130807
  Terminator1 : Terminator
  accumulator : uplink_4c1r_accumulator/accumulator  Latency=0
      link override ChannelOut: latency=4
  carrier_separation : Subsystem
  peak_detector : uplink_4c1r_peak_detector/peak_detector  Latency=0
      link override ChannelOut: latency=1
  wires:
  carrier_separation/4(pulse_1ms_out) -> peak_detector/4, accumulator/4
  Reg_busy_bit/1 -> Reg_Block/4
  Scale/3 -> peak_detector/3, accumulator/3
  Scale/2 -> peak_detector/2, accumulator/2
  Scale/1 -> peak_detector/1, accumulator/1
  peak_detector/2 -> Reg_Block/3
  accumulator/1 -> Reg_Block/2
  peak_detector/1 -> Reg_Block/1
  carrier_separation/1("axc1_data_out ") -> Scale/1
  Const/1 -> Scale/4
  valid/1 -> carrier_separation/1(valid)
  channel/1 -> carrier_separation/2(channel)
  "data "/1 -> carrier_separation/3("data ")
  Scale/4 -> Terminator1/1
  pulse_1msec/1 -> carrier_separation/4("1ms_pulse_in ")
  carrier_separation/2(valid_out) -> Scale/2
  carrier_separation/3(channel_out) -> Scale/3

== system uplink_4c1r/DUT/Power_Meter_ddc_out ==
  v : Inport
  c : Inport  Port=2
  d : Inport  Port=3
  pulse_in : Inport  Port=4
  Reg_sync_Bit : Inport  Port=5
  Carrier1 : Subsystem  AncestorBlock=uplink_4c1r_pd_accu_reg_block/Subsystem  mask{Peak_Detector_address=power_meter_param.ddc_carr1_out_pd_address, Accumulator1_addr=power_meter_param.ddc_carr1_out_acc1_reg_addr, Accumulator2_addr=power_meter_param.ddc_carr1_out_acc2_reg_addr, Latency=20}
      mask Display:
      | disp('PD_ACCU_REG_BLOCK');
      | port_label('input',1,'d');
      | port_label('input',2,'v');
      | port_label('input',3,'c');
      | port_label('input',4,'pulse_in');
      | port_label('input',5,'Reg_Busy_Bit');
  Carrier2 : Subsystem  AncestorBlock=uplink_4c1r_pd_accu_reg_block/Subsystem  mask{Peak_Detector_address=power_meter_param.ddc_carr2_out_pd_address, Accumulator1_addr=power_meter_param.ddc_carr2_out_acc1_reg_addr, Accumulator2_addr=power_meter_param.ddc_carr2_out_acc2_reg_addr, Latency=20}
      mask Display:
      | disp('PD_ACCU_REG_BLOCK');
      | port_label('input',1,'d');
      | port_label('input',2,'v');
      | port_label('input',3,'c');
      | port_label('input',4,'pulse_in');
      | port_label('input',5,'Reg_Busy_Bit');
  Carrier3 : Subsystem  AncestorBlock=uplink_4c1r_pd_accu_reg_block/Subsystem  mask{Peak_Detector_address=power_meter_param.ddc_carr3_out_pd_address, Accumulator1_addr=power_meter_param.ddc_carr3_out_acc1_reg_addr, Accumulator2_addr=power_meter_param.ddc_carr3_out_acc2_reg_addr, Latency=0}
      mask Display:
      | disp('PD_ACCU_REG_BLOCK');
      | port_label('input',1,'d');
      | port_label('input',2,'v');
      | port_label('input',3,'c');
      | port_label('input',4,'pulse_in');
      | port_label('input',5,'Reg_Busy_Bit');
  Carrier4 : Subsystem  AncestorBlock=uplink_4c1r_pd_accu_reg_block/Subsystem  mask{Peak_Detector_address=power_meter_param.ddc_carr4_out_pd_address, Accumulator1_addr=power_meter_param.ddc_carr4_out_acc1_reg_addr, Accumulator2_addr=power_meter_param.ddc_carr4_out_acc2_reg_addr, Latency=20}
      mask Display:
      | disp('PD_ACCU_REG_BLOCK');
      | port_label('input',1,'d');
      | port_label('input',2,'v');
      | port_label('input',3,'c');
      | port_label('input',4,'pulse_in');
      | port_label('input',5,'Reg_Busy_Bit');
  carrier_separation : Subsystem  AncestorBlock=uplink_4c1r_carrier_seperation_4c/carrier_separation  mask{Latency=20}
      mask Display:
      | disp('CARRIER_SEPERATION');
      | port_label('input',1,'v');
      | port_label('input',2,'c');
      | port_label('input',3,'d');
      | port_label('input',4,'pulse_in');
      | port_label('output',1,'q_carr1');
      | port_label('output',2,'qv_carr1');
      | port_label('output',3,'q_carr2');
      | port_label('output',4,'qv_carr2');
      | port_label('output',5,'q_carr3');
      | port_label('output',6,'qv_carr3');
      | port_label('output',7,'q_carr4');
      | port_label('output',8,'qv_carr4');
      | port_label('output',9,'qc');
      | port_label('output',10,'q_pulse');
  wires:
  pulse_in/1 -> carrier_separation/4("1ms_pulse_in ")
  v/1 -> carrier_separation/1(valid)
  c/1 -> carrier_separation/2(channel)
  d/1 -> carrier_separation/3("data ")
  carrier_separation/1("axc0_data_out ") -> Carrier1/1(a)
  carrier_separation/2(axc0_valid_out) -> Carrier1/2(v)
  carrier_separation/3(axc1_data_out) -> Carrier2/1(a)
  carrier_separation/4(axc1_valid_out) -> Carrier2/2(v)
  carrier_separation/5(axc2_data_out) -> Carrier3/1(a)
  carrier_separation/6(axc2_valid_out) -> Carrier3/2(v)
  carrier_separation/7(axc3_data_out) -> Carrier4/1(a)
  carrier_separation/8(axc3_valid_out) -> Carrier4/2(v)
  carrier_separation/9(channel_out) -> Carrier1/3(c), Carrier2/3(c), Carrier3/3(c), Carrier4/3(c)
  carrier_separation/10(1ms_pulse_out) -> Carrier1/4(Pulse_In), Carrier2/4(Pulse_In), Carrier3/4(Pulse_In), Carrier4/4(Pulse_In)
  Reg_sync_Bit/1 -> Carrier3/5(Reg_Busy_Bit), Carrier2/5(Reg_Busy_Bit), Carrier1/5(Reg_Busy_Bit), Carrier4/5(Reg_Busy_Bit)

== system uplink_4c1r/DUT/ddc_out_capture_rfp ==
  GPOut : DSPBAPrim/GPOut  primtype=gpout  nInputs=evalAionMaskParam(gcb,'value',1)  nOutputs=evalAionMaskParam(gcb,'value',1)  omode=Inherit via internal rule  otype=sfix(16)  scale=2^-15  rndmethod=Unbiased  factor=1  satmethod=Symmetric  shift_vec=[0 1 2 -1]  value=1  inPortNames=[' ' ' ' ' ' ' ' ' ' ' ' ' ' ' ' ' ' ' ' ' ' ' ' ' ' ' ' ' ' ' ' ' ' ' ' ' ' ' ' ' ' ' ' ' ' ' ' ' ' ' ' ' ' ' ' ' ' ' ' ' ' ' ' ' ' ' ' ' ']'  outPortNames=[' ' ' ' ' ' ' ' ' ' ' ' ' ' ' ' ' ' ' ' ' ' ' ' ' ' ' ' ' ' ' ' ' ' ' ' ' ' ' ' ' ' ' ' ' ' ' ' ' ' ' ' ' ' ' ' ' ' ' ' ' ' ' ' ' ' ' ' ' ']'  dspbaimage=dspba_prim.jpg  text=fprintf('GPOut');  style=Optimised  visibilities=1024  latencyCorrection=0  version=20090407
  SynthesisInfo : DSPBAPrim/SynthesisInfo  primtype=synthinfo  nInputs=0  nOutputs=0  omode=Inherit via internal rule  otype=sfix(16)  scale=2^-15  rndmethod=Truncate  factor=1  satmethod=Symmetric  shift_vec=[0 1 2 -1]  value=99  inPortNames=[' '; ' ';]  outPortNames=[' ']  dspbaimage=dspba_prim_ctrl.jpg  text=fprintf('Style=%s', style);  style=Scheduled  visibilities=2^15+2^17+2^18+2^19  constraintInUse=off  constraintRelation=>  constraintLimit=2  bitAccurate=off  version=20150220
  zero_idx1 : DSPBAPrim/Const  primtype=const  nInputs=0  nOutputs=1  omode=boolean  otype=ufix(1)  scale=0  rndmethod=Unbiased  factor=1  satmethod=Symmetric  shift_vec=[0 1 2 -1]  value=1  inPortNames=['+'; '+';]  outPortNames=[' ']  dspbaimage=dspba_prim.jpg  text=fprintf('%s', num2str(value));  style=Optimised  visibilities=8 + 1024  floatPrecision=float32_m23  version=20120820
  Out_RFP : Outport
  wires:
  GPOut/1 -> Out_RFP/1
  zero_idx1/1 -> GPOut/1

== system uplink_4c1r/DUT/ddc_out_rfp ==
  GPOut : DSPBAPrim/GPOut  primtype=gpout  nInputs=evalAionMaskParam(gcb,'value',1)  nOutputs=evalAionMaskParam(gcb,'value',1)  omode=Inherit via internal rule  otype=sfix(16)  scale=2^-15  rndmethod=Unbiased  factor=1  satmethod=Symmetric  shift_vec=[0 1 2 -1]  value=1  inPortNames=[' ' ' ' ' ' ' ' ' ' ' ' ' ' ' ' ' ' ' ' ' ' ' ' ' ' ' ' ' ' ' ' ' ' ' ' ' ' ' ' ' ' ' ' ' ' ' ' ' ' ' ' ' ' ' ' ' ' ' ' ' ' ' ' ' ' ' ' ' ']'  outPortNames=[' ' ' ' ' ' ' ' ' ' ' ' ' ' ' ' ' ' ' ' ' ' ' ' ' ' ' ' ' ' ' ' ' ' ' ' ' ' ' ' ' ' ' ' ' ' ' ' ' ' ' ' ' ' ' ' ' ' ' ' ' ' ' ' ' ' ' ' ' ']'  dspbaimage=dspba_prim.jpg  text=fprintf('GPOut');  style=Optimised  visibilities=1024  latencyCorrection=0  version=20090407
  SynthesisInfo : DSPBAPrim/SynthesisInfo  primtype=synthinfo  nInputs=0  nOutputs=0  omode=Inherit via internal rule  otype=sfix(16)  scale=2^-15  rndmethod=Truncate  factor=1  satmethod=Symmetric  shift_vec=[0 1 2 -1]  value=99  inPortNames=[' '; ' ';]  outPortNames=[' ']  dspbaimage=dspba_prim_ctrl.jpg  text=fprintf('Style=%s', style);  style=Scheduled  visibilities=2^15+2^17+2^18+2^19  constraintInUse=off  constraintRelation=>  constraintLimit=2  bitAccurate=off  version=20150220
  zero_idx1 : DSPBAPrim/Const  primtype=const  nInputs=0  nOutputs=1  omode=boolean  otype=ufix(1)  scale=0  rndmethod=Unbiased  factor=1  satmethod=Symmetric  shift_vec=[0 1 2 -1]  value=1  inPortNames=['+'; '+';]  outPortNames=[' ']  dspbaimage=dspba_prim.jpg  text=fprintf('%s', num2str(value));  style=Optimised  visibilities=8 + 1024  floatPrecision=float32_m23  version=20120820
  Out_RFP : Outport
  wires:
  zero_idx1/1 -> GPOut/1
  GPOut/1 -> Out_RFP/1

== system uplink_4c1r/DUT/input_capture_rfp ==
  GPOut : DSPBAPrim/GPOut  primtype=gpout  nInputs=evalAionMaskParam(gcb,'value',1)  nOutputs=evalAionMaskParam(gcb,'value',1)  omode=Inherit via internal rule  otype=sfix(16)  scale=2^-15  rndmethod=Unbiased  factor=1  satmethod=Symmetric  shift_vec=[0 1 2 -1]  value=1  inPortNames=[' ' ' ' ' ' ' ' ' ' ' ' ' ' ' ' ' ' ' ' ' ' ' ' ' ' ' ' ' ' ' ' ' ' ' ' ' ' ' ' ' ' ' ' ' ' ' ' ' ' ' ' ' ' ' ' ' ' ' ' ' ' ' ' ' ' ' ' ' ']'  outPortNames=[' ' ' ' ' ' ' ' ' ' ' ' ' ' ' ' ' ' ' ' ' ' ' ' ' ' ' ' ' ' ' ' ' ' ' ' ' ' ' ' ' ' ' ' ' ' ' ' ' ' ' ' ' ' ' ' ' ' ' ' ' ' ' ' ' ' ' ' ' ']'  dspbaimage=dspba_prim.jpg  text=fprintf('GPOut');  style=Optimised  visibilities=1024  latencyCorrection=0  version=20090407
  SynthesisInfo : DSPBAPrim/SynthesisInfo  primtype=synthinfo  nInputs=0  nOutputs=0  omode=Inherit via internal rule  otype=sfix(16)  scale=2^-15  rndmethod=Truncate  factor=1  satmethod=Symmetric  shift_vec=[0 1 2 -1]  value=99  inPortNames=[' '; ' ';]  outPortNames=[' ']  dspbaimage=dspba_prim_ctrl.jpg  text=fprintf('Style=%s', style);  style=Scheduled  visibilities=2^15+2^17+2^18+2^19  constraintInUse=off  constraintRelation=>  constraintLimit=2  bitAccurate=off  version=20150220
  zero_idx1 : DSPBAPrim/Const  primtype=const  nInputs=0  nOutputs=1  omode=boolean  otype=ufix(1)  scale=0  rndmethod=Unbiased  factor=1  satmethod=Symmetric  shift_vec=[0 1 2 -1]  value=1  inPortNames=['+'; '+';]  outPortNames=[' ']  dspbaimage=dspba_prim.jpg  text=fprintf('%s', num2str(value));  style=Optimised  visibilities=8 + 1024  floatPrecision=float32_m23  version=20120820
  Out_RFP : Outport
  wires:
  GPOut/1 -> Out_RFP/1
  zero_idx1/1 -> GPOut/1

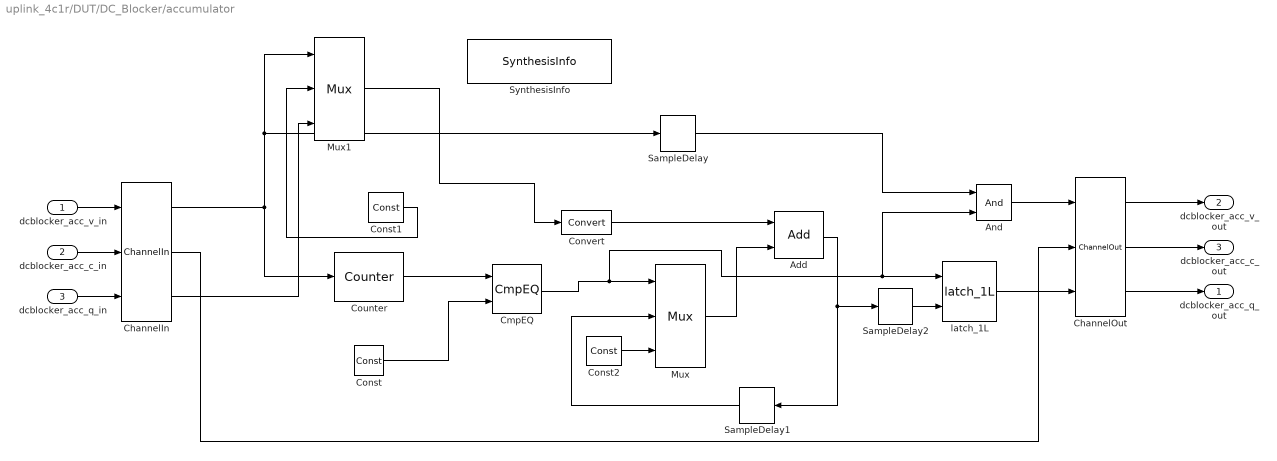
== system uplink_4c1r/DUT/DC_Blocker/accumulator ==
  dcblocker_acc_v_in : Inport
  dcblocker_acc_c_in : Inport  Port=2
  dcblocker_acc_q_in : Inport  Port=3
  Add : DSPBAPrim/Add  primtype=add  nInputs=evalAionMaskParam(gcb,'value',1)  nOutputs=1  omode=Specify via dialog  otype=sfix(24)  scale=2^-15  rndmethod=Unbiased  factor=1  satmethod=Symmetric  shift_vec=[0 1 2 -1]  value=2  inPortNames=[' '; ' ';]  outPortNames=[' ']  dspbaimage=dspba_prim.jpg  text=fprintf('+');  style=Optimised  visibilities=1032+2^17+2^18+2^19  genFPC=off  floatRounding=correct  advOptions=[]  version=20130821
  And : DSPBAPrim/And  primtype=and  nInputs=2  nOutputs=1  omode=Inherit via internal rule  otype=sfix(16)  scale=2^-15  rndmethod=Unbiased  factor=1  satmethod=Symmetric  shift_vec=[0 1 2 -1]  value=0  inPortNames=[' '; ' '; ' '; ' '; ' '; ' '; ' '; ' '; ' '; ' '; ' '; ' '; ' '; ' '; ' '; ' '; ]  outPortNames=[' ']  dspbaimage=dspba_prim.jpg  text=fprintf('&');  style=Optimised  visibilities=8+2  version=20090407
  ChannelIn : DSPBAPrim/ChannelIn  primtype=channelin  nInputs=dspba_internal_get_channel_ports(gcb)  nOutputs=dspba_internal_get_channel_ports(gcb)  omode=Inherit via internal rule  otype=sfix(16)  scale=2^-15  rndmethod=Unbiased  factor=1  satmethod=Symmetric  shift_vec=[0 1 2 -1]  value=1  inPortNames=['v'; 'c'; '0'; '1'; '2'; '3'; '4'; '5'; '6'; '7'; '8'; '9'; 'A'; 'B'; 'D'; 'E'; 'F'; 'G'; 'H'; 'I'; 'J'; 'K'; 'L'; 'M'; 'N'; 'O'; 'P'; 'Q'; 'R'; 'S'; 'T'; 'U'; 'W'; 'X'; 'Y'; 'Z']  outPortNames=['v'; 'c'; '0'; '1'; '2'; '3'; '4'; '5'; '6'; '7'; '8'; '9'; 'A'; 'B'; 'D'; 'E'; 'F'; 'G'; 'H'; 'I'; 'J'; 'K'; 'L'; 'M'; 'N'; 'O'; 'P'; 'Q'; 'R'; 'S'; 'T'; 'U'; 'W'; 'X'; 'Y'; 'Z']  dspbaimage=dspba_prim.jpg  text=fprintf('In');  style=Optimised  dataSignals=1  foldingEnabled=off  channels=1  sampleRate=200  packetBeginPresent=off  packetBeginEnabled=off  visibilities=dspba_ChannelInVis(gcb)  latencyCorrection=0  version=20141013
  ChannelOut : DSPBAPrim/ChannelOut  primtype=channelout  nInputs=dspba_internal_get_channel_ports(gcb)  nOutputs=dspba_internal_get_channel_ports(gcb)  omode=Inherit via internal rule  otype=sfix(16)  scale=2^-15  rndmethod=Unbiased  factor=1  satmethod=Symmetric  shift_vec=[0 1 2 -1]  value=1  inPortNames=['v'; 'c'; '0'; '1'; '2'; '3'; '4'; '5'; '6'; '7'; '8'; '9'; 'A'; 'B'; 'D'; 'E'; 'F'; 'G'; 'H'; 'I'; 'J'; 'K'; 'L'; 'M'; 'N'; 'O'; 'P'; 'Q'; 'R'; 'S'; 'T'; 'U'; 'W'; 'X'; 'Y'; 'Z']  outPortNames=['v'; 'c'; '0'; '1'; '2'; '3'; '4'; '5'; '6'; '7'; '8'; '9'; 'A'; 'B'; 'D'; 'E'; 'F'; 'G'; 'H'; 'I'; 'J'; 'K'; 'L'; 'M'; 'N'; 'O'; 'P'; 'Q'; 'R'; 'S'; 'T'; 'U'; 'W'; 'X'; 'Y'; 'Z']  dspbaimage=dspba_prim.jpg  text=fprintf('Out%s', AdvDSPBChannelOutDisplay(latency));  style=Optimised  dataSignals=1  foldingEnabled=off  channels=1  sampleRate=200  packetBeginPresent=off  packetBeginEnabled=off  visibilities=dspba_ChannelOutVis(gcb)  latency=21  latencyCorrection=0  version=20141013
  CmpEQ : DSPBAPrim/CmpEQ  primtype=cmpeq  nInputs=2  nOutputs=1  omode=boolean  otype=sfix(16)  scale=2^-15  rndmethod=Unbiased  factor=1  satmethod=Symmetric  shift_vec=[0 1 2 -1]  value=0  inPortNames=[' '; ' ';]  outPortNames=[' ']  dspbaimage=dspba_prim.jpg  text=fprintf('==');  style=Optimised  visibilities=0  advOptions=[]  version=20130117
  Const : DSPBAPrim/Const  primtype=const  nInputs=0  nOutputs=1  omode=Specify via dialog  otype=uint(8)  scale=0  rndmethod=Unbiased  factor=1  satmethod=Symmetric  shift_vec=[0 1 2 -1]  value=255  inPortNames=['+'; '+';]  outPortNames=[' ']  dspbaimage=dspba_prim.jpg  text=fprintf('%s', num2str(value));  style=Optimised  visibilities=8 + 1024  floatPrecision=float32_m23  version=20120820
  Const1 : DSPBAPrim/Const  primtype=const  nInputs=0  nOutputs=1  omode=Specify via dialog  otype=sfix(16)  scale=2^-15  rndmethod=Unbiased  factor=1  satmethod=Symmetric  shift_vec=[0 1 2 -1]  value=0  inPortNames=['+'; '+';]  outPortNames=[' ']  dspbaimage=dspba_prim.jpg  text=fprintf('%s', num2str(value));  style=Optimised  visibilities=8 + 1024  floatPrecision=float32_m23  version=20120820
  Const2 : DSPBAPrim/Const  primtype=const  nInputs=0  nOutputs=1  omode=Specify via dialog  otype=sfix(24)  scale=2^-15  rndmethod=Unbiased  factor=1  satmethod=Symmetric  shift_vec=[0 1 2 -1]  value=0  inPortNames=['+'; '+';]  outPortNames=[' ']  dspbaimage=dspba_prim.jpg  text=fprintf('%s', num2str(value));  style=Optimised  visibilities=8 + 1024  floatPrecision=float32_m23  version=20120820
  Convert : DSPBAPrim/Convert  primtype=convert  nInputs=1  nOutputs=1  omode=Specify via dialog  otype=sfix(24)  scale=2^-15  rndmethod=Unbiased  factor=1  satmethod=None  shift_vec=[0 1 2 -1]  value=round([0:255]/17)  inPortNames=[' '; ' ';]  outPortNames=[' '; 'c']  dspbaimage=dspba_prim.jpg  text=fprintf('convert');  style=Optimised  visibilities=8+64+256+2^17  clipdetect=off  floatPrecision=float32_m23  advOptions=[]  version=20130211
  Counter : DSPBAPrim/Counter  primtype=counter  nInputs=1  nOutputs=1  omode=Inherit via internal rule  otype=ufix(16)  scale=2^-0  rndmethod=Unbiased  factor=1  satmethod=Symmetric  shift_vec=[0 1 2 -1]  value=[0 256 1]  inPortNames=[' '; ' ';]  outPortNames=[' ']  dspbaimage=dspba_prim.jpg  text=fprintf('counter\n[%d %d %d]', value(1), value(2), value(3));  style=Optimised  visibilities=8 + 1024  version=20090407
  Mux : DSPBAPrim/Mux  primtype=mux  nInputs=evalAionMaskParam(gcb,'value',1)+1  nOutputs=1  omode=Inherit via internal rule  otype=sfix(16)  scale=2^-15  rndmethod=Unbiased  factor=1  satmethod=Symmetric  shift_vec=[0 1 2 -1]  value=2  inPortNames=['s'; 'd0'; 'd1'; 'd2'; 'd3'; 'd4'; 'd5'; 'd6'; 'd7'; 'd8'; 'd9';]  outPortNames=[' ']  dspbaimage=dspba_prim.jpg  text=fprintf('%s', primtype);  style=Optimised  visibilities=1032  version=20131025
  Mux1 : DSPBAPrim/Mux  primtype=mux  nInputs=evalAionMaskParam(gcb,'value',1)+1  nOutputs=1  omode=Inherit via internal rule  otype=sfix(16)  scale=2^-15  rndmethod=Unbiased  factor=1  satmethod=Symmetric  shift_vec=[0 1 2 -1]  value=2  inPortNames=['s'; 'd0'; 'd1'; 'd2'; 'd3'; 'd4'; 'd5'; 'd6'; 'd7'; 'd8'; 'd9';]  outPortNames=[' ']  dspbaimage=dspba_prim.jpg  text=fprintf('%s', primtype);  style=Optimised  visibilities=1032  version=20131025
  SampleDelay : DSPBAPrim/SampleDelay  primtype=sampdelay  nInputs=1  nOutputs=1  omode=Inherit via internal rule  otype=sfix(16)  scale=2^-15  rndmethod=Unbiased  factor=1  satmethod=Symmetric  shift_vec=[0 1 2 -1]  value=1  inPortNames=[' '; ' ';]  outPortNames=[' ']  dspbaimage=dspba_prim.jpg  text=dpoly(1, eye(1,value+1), 'z')  style=Optimised  visibilities=8 + 1024 + 2^17 + 2^18  flexible=off  slackgroup=0  augmented=0  version=20090407  advOptions=[]
  SampleDelay1 : DSPBAPrim/SampleDelay  primtype=sampdelay  nInputs=1  nOutputs=1  omode=Inherit via internal rule  otype=sfix(16)  scale=2^-15  rndmethod=Unbiased  factor=1  satmethod=Symmetric  shift_vec=[0 1 2 -1]  value=1  inPortNames=[' '; ' ';]  outPortNames=[' ']  dspbaimage=dspba_prim.jpg  text=dpoly(1, eye(1,value+1), 'z')  style=Optimised  visibilities=8 + 1024 + 2^17 + 2^18  flexible=off  slackgroup=0  augmented=0  version=20090407  advOptions=[]
  SampleDelay2 : DSPBAPrim/SampleDelay  primtype=sampdelay  nInputs=1  nOutputs=1  omode=Inherit via internal rule  otype=sfix(16)  scale=2^-15  rndmethod=Unbiased  factor=1  satmethod=Symmetric  shift_vec=[0 1 2 -1]  value=1  inPortNames=[' '; ' ';]  outPortNames=[' ']  dspbaimage=dspba_prim.jpg  text=dpoly(1, eye(1,value+1), 'z')  style=Optimised  visibilities=8 + 1024 + 2^17 + 2^18  flexible=off  slackgroup=0  augmented=0  version=20090407  advOptions=[]
  SynthesisInfo : DSPBAPrim/SynthesisInfo  primtype=synthinfo  nInputs=0  nOutputs=0  omode=Inherit via internal rule  otype=sfix(16)  scale=2^-15  rndmethod=Truncate  factor=1  satmethod=Symmetric  shift_vec=[0 1 2 -1]  value=99  inPortNames=[' '; ' ';]  outPortNames=[' ']  dspbaimage=dspba_prim_ctrl.jpg  text=fprintf('Style=%s', style);  style=Scheduled  visibilities=2^15+2^17+2^18+2^19  constraintInUse=on  constraintRelation=>  constraintLimit=20  bitAccurate=off  version=20150220
  latch_1L : DSPBAControl/latch_1L
  dcblocker_acc_q_out : Outport
  dcblocker_acc_v_out : Outport  Port=2
  dcblocker_acc_c_out : Outport  Port=3
  wires:
  Const/1 -> CmpEQ/2
  Counter/1 -> CmpEQ/1
  ChannelIn/1 -> SampleDelay/1, Mux1/1, Counter/1
  ChannelIn/3 -> Mux1/3
  dcblocker_acc_c_in/1 -> ChannelIn/2
  dcblocker_acc_v_in/1 -> ChannelIn/1
  dcblocker_acc_q_in/1 -> ChannelIn/3
  ChannelIn/2 -> ChannelOut/2
  ChannelOut/1 -> dcblocker_acc_v_out/1
  ChannelOut/3 -> dcblocker_acc_q_out/1
  ChannelOut/2 -> dcblocker_acc_c_out/1
  Mux1/1 -> Convert/1
  Mux/1 -> Add/2
  Add/1 -> SampleDelay2/1, SampleDelay1/1
  Convert/1 -> Add/1
  SampleDelay1/1 -> Mux/2
  Const1/1 -> Mux1/2
  SampleDelay/1 -> And/1
  Const2/1 -> Mux/3
  latch_1L/1 -> ChannelOut/3
  CmpEQ/1 -> And/2, latch_1L/1, Mux/1
  SampleDelay2/1 -> latch_1L/2
  And/1 -> ChannelOut/1
